simulink model "SEPIC_SIMU"  (R2017b)
settings: Solver=ode23t  StartTime=0.0  StopTime=0.2  MaxStep=100e-9  RelTol=100e-9
values from neighbouring files (symbols this model uses):
  Aramp = -(Ma*Ts)    (= 0.37875)    [PLANT STABILITY.m]    (also in PLANT_STABILITY.m = -(Ma*Ts))
  C = 56*10^-6    (= 5.6e-05)    [CODIGO_MATLAB_PLANTA_ESTABILIDAD_CONTROLADOR.m]    (also in PLANT STABILITY.m; PLANT_STABILITY.m)
  CIN = 56*10^-6    (= 5.6e-05)    [CODIGO_MATLAB_PLANTA_ESTABILIDAD_CONTROLADOR.m]    (also in PLANT STABILITY.m; PLANT_STABILITY.m)
  CX = 56*10^-6    (= 5.6e-05)    [CODIGO_MATLAB_PLANTA_ESTABILIDAD_CONTROLADOR.m]    (also in PLANT STABILITY.m; PLANT_STABILITY.m)
  ESR = 0.029    [CODIGO_MATLAB_PLANTA_ESTABILIDAD_CONTROLADOR.m]    (also in PLANT STABILITY.m; PLANT_STABILITY.m)
  H = 0.4640    (= 0.464)    [CODIGO_MATLAB_PLANTA_ESTABILIDAD_CONTROLADOR.m]    (also in PLANT STABILITY.m; PLANT_STABILITY.m)
  L = 220*10^-6    (= 0.00022)    [CODIGO_MATLAB_PLANTA_ESTABILIDAD_CONTROLADOR.m]    (also in PLANT STABILITY.m; PLANT_STABILITY.m)
  RSH = 0.1    [CODIGO_MATLAB_PLANTA_ESTABILIDAD_CONTROLADOR.m]    (also in PLANT STABILITY.m; PLANT_STABILITY.m)
  Td = (LimH)*Ts    [PLANT_STABILITY.m]
  Ts = 1/f    (= 1e-05)    [CODIGO_MATLAB_PLANTA_ESTABILIDAD_CONTROLADOR.m]    (also in PLANT STABILITY.m; PLANT_STABILITY.m)
  VO = 14.7    [CODIGO_MATLAB_PLANTA_ESTABILIDAD_CONTROLADOR.m]    (also in PLANT STABILITY.m; PLANT_STABILITY.m)
undefined symbols (not defined in the file or in its folder): Acid, DiscIntNeverNeededParam, Ki, Kp, Lead
libraries: powerlib x29, simulink_extras x2, powerlib_meascontrol x2, electricdrivelib x1, re_lib x1
settings Model: Creator=TG1748  LastModifiedBy=arman
settings SolverCC: ZeroCrossAlgorithm=Adaptive
settings DebuggingCC: UnconnectedInputMsg=none  UnconnectedOutputMsg=none  UnconnectedLineMsg=none
settings ConfigComp: PLC_TargetIDE=codesys23  PLC_GenerateReport=off  PLC_LaunchReport=off

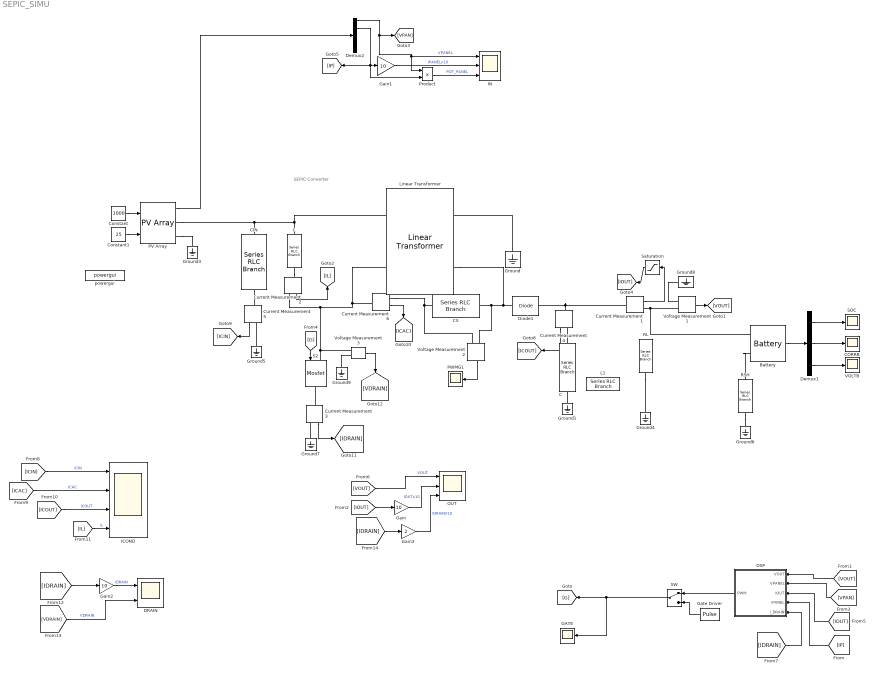
== system SEPIC_SIMU ==
  note: SEPIC Converter
  Battery : electricdrivelib/Extra Sources/Battery  BatType=Lead-Acid  ShowTempParam=off  ThermalPreset=no  ShowAgeParam=off  NomV=12  NomQ=7.2  SOC=50  Batt_Tr=30  PresetModel=off  MaxQ=7.5  MinV=9  FullV=14.7  Dis_rate=0.375  R=0.024  Normal_OP=6  expZone="[12.8        0.024]"  current=[0.375 0.746 1.32]  Units=Time  Tci=20  NomT=20  T2=-30  MaxQ2=4.8  FullV2=7.1  Normal_OP2=5.655  expZone2="[6.58           1]"  Rca=0.6  ti=2000  Dp=0  Neq0=0  Tsim=1e6  Ta1=25  Qeol=5.4*0.9  Reol=0.013333*1.2  Char_age=[2.3478, 3]  Dis_age=[2.3478, 10]  N1=1500  N2=10500  N3=1000  N4=1400  Ta2=45  N5=950
  C : powerlib/Elements/Series RLC Branch  LConnTagsString=__new0  RConnTagsString=__new0  BranchType=RC  Resistance=ESR  Inductance=1e-3  SetiL0=off  InitialCurrent=0  Capacitance=C  Setx0=off  InitialVoltage=0  Measurements=None
  CIN : powerlib/Elements/Series RLC Branch  LConnTagsString=__new0  RConnTagsString=__new0  BranchType=RC  Resistance=ESR  Inductance=1e-3  SetiL0=off  InitialCurrent=0  Capacitance=CIN  Setx0=off  InitialVoltage=0  Measurements=None
  CORRB : Scope
  CX : powerlib/Elements/Series RLC Branch  LConnTagsString=__new0  RConnTagsString=__new0  BranchType=RC  Resistance=ESR  Inductance=1e-3  SetiL0=off  InitialCurrent=0  Capacitance=CX  Setx0=off  InitialVoltage=0  Measurements=None
  Constant : Constant  Value=1000
  Constant1 : Constant  Value=25
  Current Measurement{1..6} (6 alike) : powerlib/Measurements/Current Measurement  PhasorSimulation=off  OutputType=Complex  PSBequivalent=0
  DRAIN : Scope  NumInputPorts=2
  DSP : Subsystem
  Demux1 : Demux  Outputs=3
  Demux2 : Demux  Outputs=5
  Diode1 : powerlib/Power Electronics/Diode  Ron=0.001  Lon=0  Vf=VD  IC=0  UseSnubber=off  Rs=inf  Cs=250e-9  Measurements=off
  GATE : Scope
  Gain : Gain  Gain=10
  Gain1 : Gain  Gain=10
  Gain2 : Gain  Gain=10
  Gain3 : Gain  Gain=2
  Gate Driver : DiscretePulseGenerator  PulseType=Time based  Period=Ts  PulseWidth=H*100
  Ground{,1,3..9} (9 alike) : powerlib/Elements/Ground  LConnTagsString=a
  ICOND : Scope  NumInputPorts=4
  IN : Scope  NumInputPorts=3
  L : powerlib/Elements/Series RLC Branch  LConnTagsString=__new0  RConnTagsString=__new0  BranchType=L  Resistance=1  Inductance=L  SetiL0=off  InitialCurrent=0  Capacitance=1e-6  Setx0=off  InitialVoltage=0  Measurements=None
  L1 : powerlib/Elements/Series RLC Branch  LConnTagsString=__new0  RConnTagsString=__new0  BranchType=L  Resistance=1  Inductance=3.3e-6  SetiL0=off  InitialCurrent=0  Capacitance=1e-6  Setx0=off  InitialVoltage=0  Measurements=None
  Linear Transformer : powerlib/Elements/Linear Transformer  UNITS=SI  NominalPower=[ 22 100000 ]  winding1=[1 0 0]  winding2=[1 0 0]  ThreeWindings=off  winding3=[3.15e+05 0.7938 0.084225]  RmLm=[1e6 inf]  Measurements=None  DataType=on
  OUT : Scope  NumInputPorts=3
  PV Array : re_lib/Solar/PV Array  Npar=1  Nser=1  PlotType=array @ 25 deg.C & specified irradiances  S_vec="[ 1000  500  100 ]"  Temp_C_vec="[ 45 25  ]"  ModuleName=User-defined  PlotWhenSelected=off  Pm=19.95  Ncell=36  Voc=21.6  Isc=1.23  Vm=17.5  Im=1.14  beta_Voc_pc=-0.333  alpha_Isc_pc=0.05  beta_Voc=-0.071928  alpha_Isc=0.000615  IL=1.239  I0=1.5415e-11  nI=0.93147  Rsh=462.7836  Rs=1.3323  BAL=on  Tc=1e-6  Tfilter=5e-5
  PWMG1 : Scope
  Product : Product
  RL : powerlib/Elements/Series RLC Branch  LConnTagsString=__new0  RConnTagsString=__new0  BranchType=R  Resistance=VO  Inductance=1e-3  SetiL0=off  InitialCurrent=0  Capacitance=1e-6  Setx0=off  InitialVoltage=0  Measurements=None
  RSH : powerlib/Elements/Series RLC Branch  LConnTagsString=__new0  RConnTagsString=__new0  BranchType=R  Resistance=RSH  Inductance=1e-3  SetiL0=off  InitialCurrent=0  Capacitance=1e-6  Setx0=off  InitialVoltage=0  Measurements=None
  S2 : powerlib/Power Electronics/Mosfet  Ron=0.007  Lon=0  Rd=0.0062  Vfd=1.3  IC=0  Rs=1e5  Cs=inf  Measurements=off
  SOC : Scope
  SW : ManualSwitch
  Saturation : Saturate  UpperLimit=1.5  LowerLimit=0
  VOLTB : Scope
  Voltage Measurement1 : powerlib/Measurements/Voltage Measurement  PhasorSimulation=off  OutputType=Complex  PSBequivalent=0
  Voltage Measurement2 : powerlib/Measurements/Voltage Measurement  PhasorSimulation=off  OutputType=Complex  PSBequivalent=0
  Voltage Measurement3 : powerlib/Measurements/Voltage Measurement  PhasorSimulation=off  OutputType=Complex  PSBequivalent=0
  powergui : powerlib/powergui  SimulationMode=Continuous  SampleTime=50e-6  frequency=60  Iterations=50  frequencyindice=0  Pbase=100e6  ErrMax=1e-4  UnitsV=kV  UnitsW=MW  buscounter=0  FunctionMessages=off  echomessages=off  EnableUseOfTLC=off  CurrentSourceSwitches=off  DisableSnubberDevices=off  DisableRonSwitches=off  DisableVfSwitches=off  DisplayEquations=off  SolverType=Tustin/Backward Euler (TBE)  Interpol=off  ExternalGateDelay=off  methode=off  Ts=100  x0status=blocks  SPID=on  SwTol=0  HookPort=off  RestoreLinks=warning  ResistiveCurrentMeasurement=off  Frange=[0:2:500]  Ylog=off  Xlog=on  ShowGrid=off  save=off  variable=ZData  structure=0  ZoomFFT=on  StartTime=0.0  cycles=1  DisplayStyle=1  fundamental=60  FreqAxis=off  MaxFrequency=1000  frequencyindicesteady=1  RmsSteady=1  display=off
  wires:
  Constant/1 -> PV Array/1
  Constant1/1 -> PV Array/2
  [VOUT] -> DSP/1(VOUT)
  [VPAN] -> DSP/2(VPANEL)
  Gate Driver/1 -> SW/2
  DSP/1("PWM ") -> SW/1
  [IOUT] -> DSP/3(IOUT)
  Battery/1 -> Demux1/1
  Demux1/1 -> SOC/1
  Demux1/2 -> CORRB/1
  Demux1/3 -> VOLTB/1
  PV Array/1 -> Demux2/1
  [IP] -> DSP/4(IPANEL)
  Current Measurement2/1 -> [IL]
  Voltage Measurement1/1 -> [VOUT]
  [VOUT] -> OUT/1  "VOUT"
  [IOUT] -> Gain/1
  Gain/1 -> OUT/2  "IOUTx10"
  Demux2/1 -> [VPAN], IN/1, Product/1  "VPANEL"
  Product/1 -> IN/3  "POT_PANEL"
  [IDRAIN] -> DSP/5(I_DRAIN)
  SW/1 -> GATE/1, [G]
  Current Measurement4/1 -> [ICOUT]
  Current Measurement5/1 -> [ICIN]
  Current Measurement6/1 -> [ICAC]
  [ICAC] -> ICOND/2  "ICAC"
  [ICOUT] -> ICOND/3  "ICOUT"
  [IL] -> ICOND/4  "IL"
  Voltage Measurement2/1 -> PWMG1/1
  Gain2/1 -> DRAIN/1  "IDRAIN"
  [IDRAIN] -> Gain2/1
  Voltage Measurement3/1 -> [VDRAIN]
  [G] -> S2/1
  [ICIN] -> ICOND/1  "ICIN"
  Demux2/2 -> [IP], Product/2, Gain1/1
  Gain1/1 -> IN/2  "IPANELx10"
  [VDRAIN] -> DRAIN/2  "VDRAIN"
  Saturation/1 -> [IOUT]
  Current Measurement1/1 -> Saturation/1
  Current Measurement3/1 -> [IDRAIN]
  [IDRAIN] -> Gain3/1
  Gain3/1 -> OUT/3  "IDRAINX10"
  connections:
  Current Measurement4/LConn1 -- Current Measurement1/LConn1 -- Diode1/RConn1
  Diode1/LConn1 -- Linear Transformer/RConn1 -- Voltage Measurement2/LConn2 -- CX/RConn1
  CIN/LConn1 -- PV Array/RConn1 -- L/LConn1 -- Linear Transformer/LConn2
  Ground/LConn1 -- Linear Transformer/RConn2
  PV Array/RConn2 -- Ground3/LConn1
  RL/RConn1 -- Ground4/LConn1
  Battery/LConn2 -- RSH/LConn1
  RSH/RConn1 -- Ground6/LConn1
  Current Measurement1/RConn1 -- Battery/LConn1 -- Voltage Measurement1/LConn1
  Ground8/LConn1 -- Voltage Measurement1/LConn2
  L/RConn1 -- Current Measurement2/LConn1
  Linear Transformer/LConn1 -- Current Measurement2/RConn1 -- S2/LConn1 -- Voltage Measurement3/LConn1 -- Current Measurement6/LConn1
  Current Measurement6/RConn1 -- Voltage Measurement2/LConn1 -- CX/LConn1
  Ground5/LConn1 -- Current Measurement5/RConn1
  CIN/RConn1 -- Current Measurement5/LConn1
  Current Measurement4/RConn1 -- C/LConn1
  Ground1/LConn1 -- C/RConn1
  Current Measurement3/LConn1 -- S2/RConn1
  Ground7/LConn1 -- Current Measurement3/RConn1
  Ground9/LConn1 -- Voltage Measurement3/LConn2

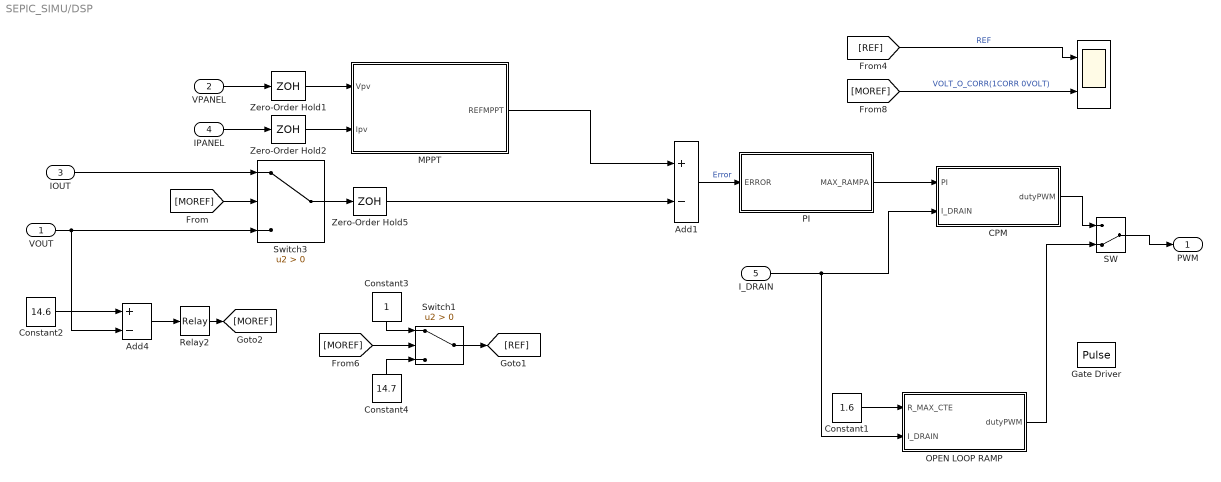
== system SEPIC_SIMU/DSP ==
  VOUT : Inport
  VPANEL : Inport  Port=2
  IOUT : Inport  Port=3
  IPANEL : Inport  Port=4
  I_DRAIN : Inport  Port=5
  " " : Scope  NumInputPorts=2
  Add1 : Sum  Inputs=+-
  Add4 : Sum  Inputs=+-
  CPM : Subsystem
  Constant1 : Constant  Value=1.6
  Constant2 : Constant  Value=14.6
  Constant3 : Constant
  Constant4 : Constant  Value=14.7
  Gate Driver : DiscretePulseGenerator  PulseType=Time based  Period=Ts  PulseWidth=H*100
  MPPT : Subsystem
  OPEN LOOP RAMP : Subsystem
  PI : Subsystem
  Relay2 : Relay  OnSwitchValue=0.1  OffSwitchValue=-0.1
  SW : ManualSwitch  CurrentSetting=0
  Switch1 : Switch  Criteria=u2 > Threshold
  Switch3 : Switch  Criteria=u2 > Threshold
  Zero-Order Hold1 : ZeroOrderHold  SampleTime=0.4e-3
  Zero-Order Hold2 : ZeroOrderHold  SampleTime=0.4e-3
  Zero-Order Hold5 : ZeroOrderHold  SampleTime=Ts
  "PWM " : Outport
  wires:
  Add1/1 -> PI/1(ERROR)  "Error"
  VOUT/1 -> Switch3/3, Add4/2
  I_DRAIN/1 -> OPEN LOOP RAMP/2(I_DRAIN), CPM/2(I_DRAIN)
  IPANEL/1 -> Zero-Order Hold2/1
  VPANEL/1 -> Zero-Order Hold1/1
  Zero-Order Hold1/1 -> MPPT/1(Vpv)
  Zero-Order Hold2/1 -> MPPT/2(Ipv)
  PI/1(MAX_RAMPA) -> CPM/1(PI)
  Switch1/1 -> [REF]
  Constant4/1 -> Switch1/3
  Constant3/1 -> Switch1/1
  Switch3/1 -> Zero-Order Hold5/1
  Constant2/1 -> Add4/1
  IOUT/1 -> Switch3/1
  [REF] -> " "/1  "REF"
  [MOREF] -> Switch3/2
  [MOREF] -> Switch1/2
  [MOREF] -> " "/2  "VOLT_O_CORR(1CORR 0VOLT)"
  Relay2/1 -> [MOREF]
  Add4/1 -> Relay2/1
  MPPT/1(REFMPPT) -> Add1/1
  Zero-Order Hold5/1 -> Add1/2
  SW/1 -> "PWM "/1
  CPM/1("\tdutyPWM ") -> SW/1
  Constant1/1 -> OPEN LOOP RAMP/1("R_MAX_CTE ")
  OPEN LOOP RAMP/1("\tdutyPWM ") -> SW/2

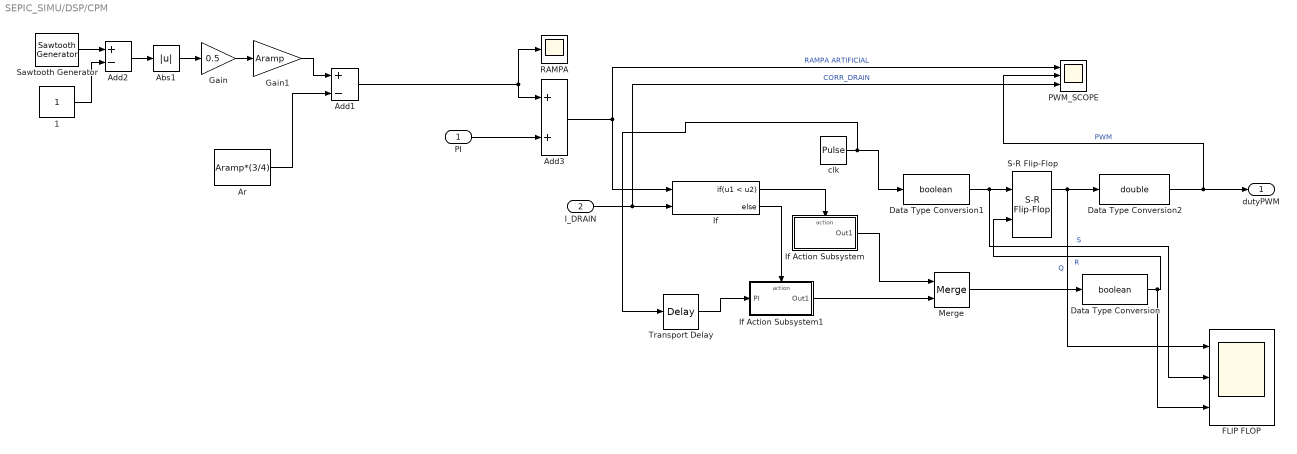
== system SEPIC_SIMU/DSP/CPM ==
  PI : Inport
  I_DRAIN : Inport  Port=2
  "1 " : Constant
  Abs1 : Abs
  Add1 : Sum  Inputs=+-
  Add2 : Sum  Inputs=+-
  Add3 : Sum
  "Ar " : Constant  Value=Aramp*(3/4)
  Data Type Conversion : DataTypeConversion  OutDataTypeStr=boolean
  Data Type Conversion1 : DataTypeConversion  OutDataTypeStr=boolean
  Data Type Conversion2 : DataTypeConversion  OutDataTypeStr=double
  "FLIP FLOP " : Scope  NumInputPorts=3
  Gain : Gain  Gain=0.5
  Gain1 : Gain  Gain=Aramp
  If : If  NumInputs=2  IfExpression=u1 < u2
  If Action Subsystem : Subsystem  TreatAsAtomicUnit=on
  If Action Subsystem1 : Subsystem  TreatAsAtomicUnit=on
  Merge : Merge
  PWM_SCOPE : Scope  NumInputPorts=3
  RAMPA : Scope
  S-R Flip-Flop : simulink_extras/Flip Flops/S-R Flip-Flop  initial_condition=0
  Sawtooth Generator : powerlib_meascontrol/Pulse & Signal Generators/Sawtooth Generator  Freq=f  Phase=0  Ts=0
      settings: SourceProductName=Simscape Power Systems
  Transport Delay : TransportDelay  DelayTime=Td
  clk : DiscretePulseGenerator  PulseType=Time based  Period=Ts
  "\tdutyPWM " : Outport
  wires:
  If Action Subsystem1/1(Out1) -> Merge/2
  If Action Subsystem/1(Out1) -> Merge/1
  Data Type Conversion1/1 -> "FLIP FLOP "/2, S-R Flip-Flop/1  "S"
  Data Type Conversion2/1 -> PWM_SCOPE/2, "\tdutyPWM "/1  "PWM"
  clk/1 -> Transport Delay/1, Data Type Conversion1/1
  Data Type Conversion/1 -> "FLIP FLOP "/3, S-R Flip-Flop/2  "R"
  I_DRAIN/1 -> PWM_SCOPE/3, If/2  "CORR_DRAIN"
  If/1 -> If Action Subsystem/Action
  S-R Flip-Flop/1 -> "FLIP FLOP "/1, Data Type Conversion2/1  "Q"
  Add3/1 -> PWM_SCOPE/1, If/1  "RAMPA ARTIFICIAL"
  If/2 -> If Action Subsystem1/Action
  PI/1 -> Add3/2
  Add1/1 -> RAMPA/1, Add3/1
  "1 "/1 -> Add2/2
  Sawtooth Generator/1 -> Add2/1
  Gain/1 -> Gain1/1
  Add2/1 -> Abs1/1
  Abs1/1 -> Gain/1
  "Ar "/1 -> Add1/2
  Gain1/1 -> Add1/1
  Merge/1 -> Data Type Conversion/1
  Transport Delay/1 -> If Action Subsystem1/1(PI)

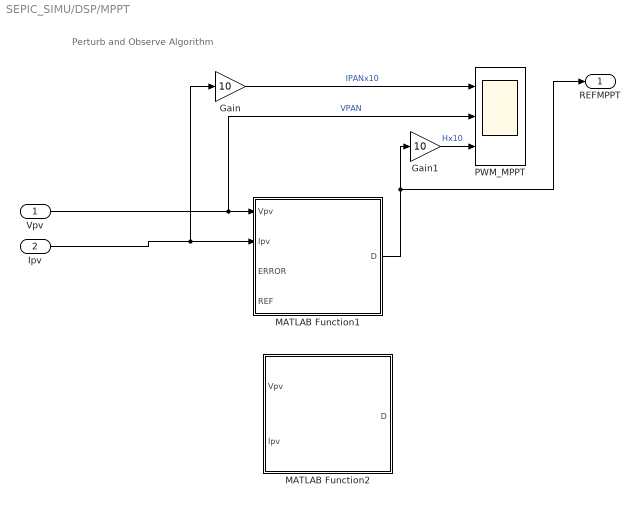
== system SEPIC_SIMU/DSP/MPPT ==
  note: Perturb and Observe Algorithm
  Vpv : Inport  OutDataTypeStr=double  PortDimensions=1  SampleTime=[0.0001,0]
  Ipv : Inport  Port=2  OutDataTypeStr=double  PortDimensions=1  SampleTime=[0.0001,0]
  Gain : Gain  Gain=10
  Gain1 : Gain  Gain=10
  MATLAB Function1 : MATLAB Function  TreatAsAtomicUnit=on  SystemSampleTime=Ts/2
  MATLAB Function2 : MATLAB Function  TreatAsAtomicUnit=on  SystemSampleTime=Ts/2
  PWM_MPPT : Scope  NumInputPorts=3
  REFMPPT : Outport  OutDataTypeStr=double  PortDimensions=1  SampleTime=[0.0001,0]
  wires:
  Vpv/1 -> MATLAB Function1/1(Vpv), PWM_MPPT/2  "VPAN"
  Ipv/1 -> MATLAB Function1/2(Ipv), Gain/1
  Gain1/1 -> PWM_MPPT/3  "Hx10"
  Gain/1 -> PWM_MPPT/1  "IPANx10"
  MATLAB Function1/1(D) -> Gain1/1, REFMPPT/1

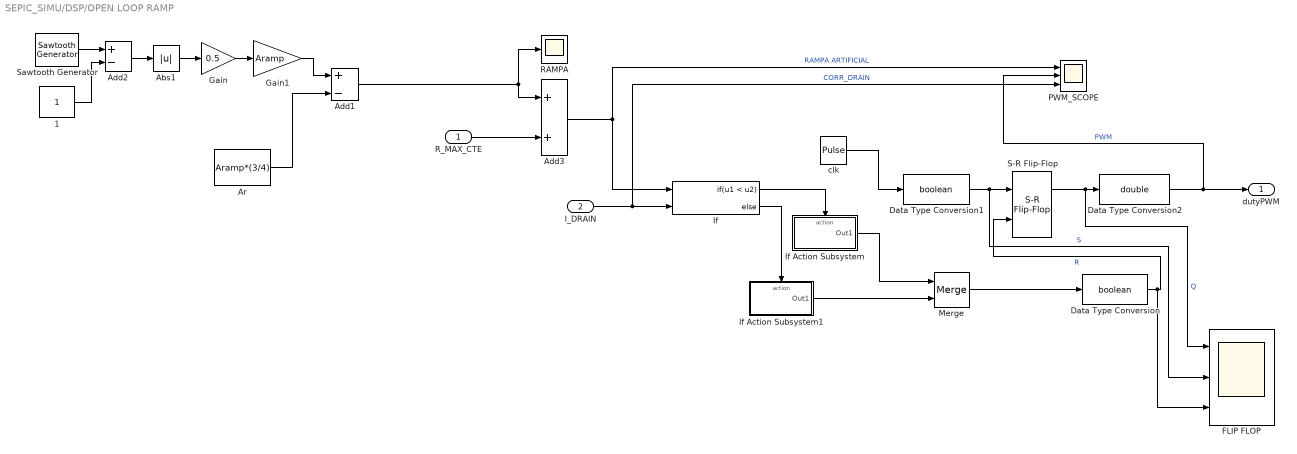
== system SEPIC_SIMU/DSP/OPEN LOOP RAMP ==
  "R_MAX_CTE " : Inport
  I_DRAIN : Inport  Port=2
  "1 " : Constant
  Abs1 : Abs
  Add1 : Sum  Inputs=+-
  Add2 : Sum  Inputs=+-
  Add3 : Sum
  "Ar " : Constant  Value=Aramp*(3/4)
  Data Type Conversion : DataTypeConversion  OutDataTypeStr=boolean
  Data Type Conversion1 : DataTypeConversion  OutDataTypeStr=boolean
  Data Type Conversion2 : DataTypeConversion  OutDataTypeStr=double
  "FLIP FLOP " : Scope  NumInputPorts=3
  Gain : Gain  Gain=0.5
  Gain1 : Gain  Gain=Aramp
  If : If  NumInputs=2  IfExpression=u1 < u2
  If Action Subsystem : Subsystem  TreatAsAtomicUnit=on
  If Action Subsystem1 : Subsystem  TreatAsAtomicUnit=on
  Merge : Merge
  PWM_SCOPE : Scope  NumInputPorts=3
  RAMPA : Scope
  S-R Flip-Flop : simulink_extras/Flip Flops/S-R Flip-Flop  initial_condition=0
  Sawtooth Generator : powerlib_meascontrol/Pulse & Signal Generators/Sawtooth Generator  Freq=f  Phase=0  Ts=0
      settings: SourceProductName=Simscape Power Systems
  clk : DiscretePulseGenerator  PulseType=Time based  Period=Ts
  "\tdutyPWM " : Outport
  wires:
  If Action Subsystem1/1(Out1) -> Merge/2
  If Action Subsystem/1(Out1) -> Merge/1
  Data Type Conversion1/1 -> "FLIP FLOP "/2, S-R Flip-Flop/1  "S"
  Data Type Conversion2/1 -> PWM_SCOPE/2, "\tdutyPWM "/1  "PWM"
  clk/1 -> Data Type Conversion1/1
  Data Type Conversion/1 -> "FLIP FLOP "/3, S-R Flip-Flop/2  "R"
  I_DRAIN/1 -> PWM_SCOPE/3, If/2  "CORR_DRAIN"
  If/1 -> If Action Subsystem/Action
  Add3/1 -> PWM_SCOPE/1, If/1  "RAMPA ARTIFICIAL"
  If/2 -> If Action Subsystem1/Action
  "R_MAX_CTE "/1 -> Add3/2
  Add1/1 -> RAMPA/1, Add3/1
  "1 "/1 -> Add2/2
  Sawtooth Generator/1 -> Add2/1
  Gain/1 -> Gain1/1
  Add2/1 -> Abs1/1
  Abs1/1 -> Gain/1
  "Ar "/1 -> Add1/2
  Gain1/1 -> Add1/1
  Merge/1 -> Data Type Conversion/1
  S-R Flip-Flop/1 -> "FLIP FLOP "/1, Data Type Conversion2/1  "Q"

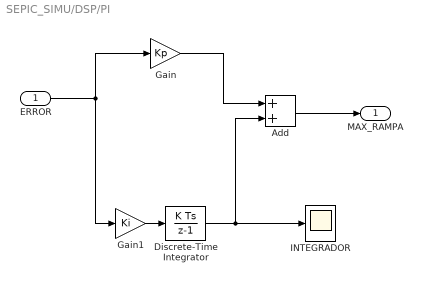
== system SEPIC_SIMU/DSP/PI ==
  ERROR : Inport
  Add : Sum
  Discrete-Time Integrator : DiscreteIntegrator  gainval=1  InitialConditionSetting=State (most efficient)  SampleTime=Ts  LimitOutput=on  UpperSaturationLimit=2.7  LowerSaturationLimit=0  ICPrevOutput=DiscIntNeverNeededParam  ICPrevScaledInput=DiscIntNeverNeededParam
  Gain : Gain  Gain=Kp
  Gain1 : Gain  Gain=Ki
  INTEGRADOR : Scope
  MAX_RAMPA : Outport
  wires:
  ERROR/1 -> Gain1/1, Gain/1
  Add/1 -> MAX_RAMPA/1
  Gain/1 -> Add/1
  Discrete-Time Integrator/1 -> Add/2, INTEGRADOR/1
  Gain1/1 -> Discrete-Time Integrator/1

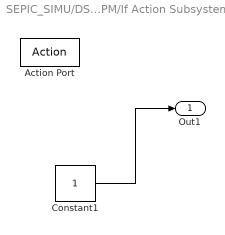
== system SEPIC_SIMU/DSP/CPM/If Action Subsystem ==
  Action Port : ActionPort  ActionType=then
  Constant1 : Constant
  Out1 : Outport
  wires:
  Constant1/1 -> Out1/1

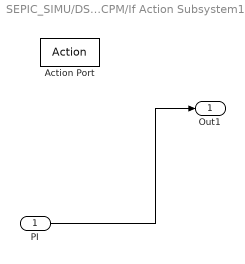
== system SEPIC_SIMU/DSP/CPM/If Action Subsystem1 ==
  PI : Inport
  Action Port : ActionPort  ActionType=else
  Out1 : Outport
  wires:
  PI/1 -> Out1/1

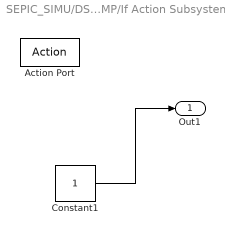
== system SEPIC_SIMU/DSP/OPEN LOOP RAMP/If Action Subsystem ==
  Action Port : ActionPort  ActionType=then
  Constant1 : Constant
  Out1 : Outport
  wires:
  Constant1/1 -> Out1/1

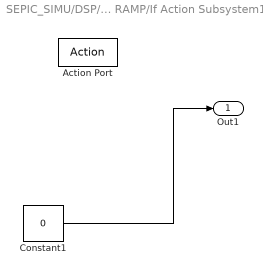
== system SEPIC_SIMU/DSP/OPEN LOOP RAMP/If Action Subsystem1 ==
  Action Port : ActionPort  ActionType=else
  Constant1 : Constant  Value=0
  Out1 : Outport
  wires:
  Constant1/1 -> Out1/1

== matlab function SEPIC_SIMU/DSP/MPPT/MATLAB Function2 ==
  data: Vpv input; D output; Ipv input
function D = CondInc(Vpv,Ipv)
% coder.extrinsic('set_param')
%#codegen
% ************************************************************
% MATLAB implementation of a Perturb and Observe algorithm
% for Maximum Power Point Tracking. This algorithm is designed
% to operate with a buck converter
%
% Created by: Carlos Osorio
% ************************************************************

% Define internal values for the voltage and power as persistent
% variables

% Pause the model
% set_param('vdp','SimulationCommand','pause');

persistent Dprev  vi ii


if isempty(Dprev)

    vi=0;
    ii=0;
    Dprev = 0.01;
    
end



deltaD = 0.001;


dv=Vpv-vi;
di=Ipv-ii;

% Increase or decrease duty cycle based on conditions
if (dv==0)
        if (di==0)
            D = Dprev;
        else
            if (di>0)
                D = Dprev-deltaD;
            else
                D = Dprev+deltaD;
            end
        end
        
    else
        if ((di/dv)==-(1.14/17.5))
            D = Dprev;
        else
            if ((di/dv)>-(1.14/17.5))
                D = Dprev-deltaD;
            else
                D = Dprev+deltaD;
            end
        end
end

vi=Vpv;
ii=Ipv;
Dprev = D;
%PREGUNTARLE A KARIM POR QUE NO SI FUNCIONA MEJOR

% if ERROR<0;
%     
%     D=Dprev;
%     
% end

== matlab function SEPIC_SIMU/DSP/MPPT/MATLAB Function1 ==
  data: Vpv input; D output; Ipv input; ERROR input; REF input
function D = PertYObs(Vpv,Ipv,ERROR,REF)
% coder.extrinsic('set_param')
%#codegen
% ************************************************************
% MATLAB implementation of a Perturb and Observe algorithm
% for Maximum Power Point Tracking. This algorithm is designed
% to operate with a buck converter
%
% Created by: Carlos Osorio
% ************************************************************

% Define internal values for the voltage and power as persistent
% variables

% Pause the model
% set_param('vdp','SimulationCommand','pause');

persistent Dprev Pprev Vprev Contbaj

% Initialize the internal values for the voltage and power on the
% first pass
if isempty(Dprev)
%     Para carga y Tm 10 ms
%     Dprev = 0.325;

    Dprev = 0.01;
% Dprev=0.1;
    Vprev = 17;
    Pprev = 0;
    
end

% Initialize algorithm parameters

deltaD = 0.001;

% deltaD = 0.01;

% Calculate measured array power
Ppv = Vpv*Ipv;

% Increase or decrease duty cycle based on conditions
if (Ppv-Pprev) ~= 0
    if (Ppv-Pprev) > 0
        if (Vpv-Vprev) > 0
            D = Dprev - deltaD;
        else
            D = Dprev + deltaD;
        end
    else
        if (Vpv-Vprev) > 0
            D = Dprev + deltaD;
        else
            D = Dprev - deltaD;
        end        
    end
else
    D = Dprev;
end

%PREGUNTARLE A KARIM POR QUE NO SI FUNCIONA MEJOR

% if ERROR<0;
%     
%     D=Dprev;
%     
% end




% Update internal values
Dprev = D;
Vprev = Vpv;
Pprev = Ppv;

% Continue
% set_param('vdp','SimulationCommand','continue');
